simulink model "mass_spring_damper"  (R2023a)
settings: Solver=VariableStepAuto  StartTime=0.0  StopTime=10.0  RelTol=1e-3
undefined symbols (not defined in the file or in its folder): c, dxdt_init, k, m, x_init
settings Model: Creator=User  LastModifiedBy=User

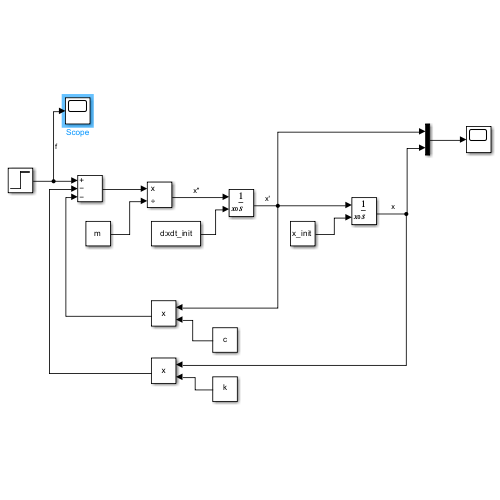
[thumbnail: Simulink's stored preview of the top-level diagram]
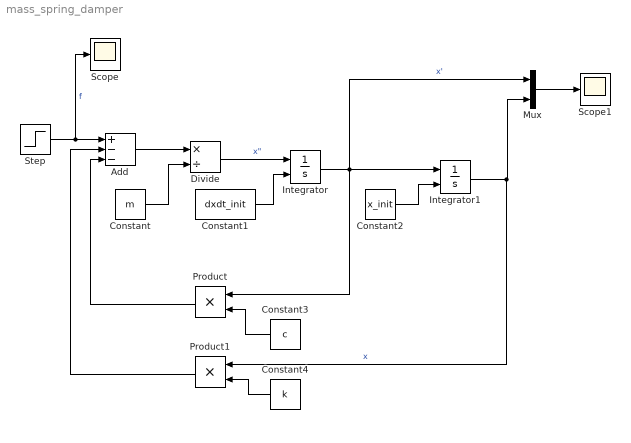
== system mass_spring_damper ==
  Add : Sum  Inputs=+--
  Constant : Constant  Value=m
  Constant1 : Constant  Value=dxdt_init  SampleTime=dxdt_init
  Constant2 : Constant  Value=x_init
  Constant3 : Constant  Value=c
  Constant4 : Constant  Value=k
  Divide : Product  Inputs=*/
  Integrator : Integrator  InitialConditionSource=external
  Integrator1 : Integrator  InitialConditionSource=external
  Mux : Mux  Inputs=2
  Product : Product
  Product1 : Product
  Scope : Scope
  Scope1 : Scope
  Step : Step  SampleTime=0
  wires:
  Step/1 -> Scope/1, Add/1  "f"
  Add/1 -> Divide/1
  Constant/1 -> Divide/2
  Divide/1 -> Integrator/1  "x\""
  Constant1/1 -> Integrator/2
  Integrator/1 -> Product/1, Mux/1, Integrator1/1  "x'"
  Constant2/1 -> Integrator1/2
  Constant3/1 -> Product/2
  Product/1 -> Add/3
  Constant4/1 -> Product1/2
  Product1/1 -> Add/2
  Mux/1 -> Scope1/1
  Integrator1/1 -> Product1/1, Mux/2  "x"
